simulink model "arduino_closed_loop_opcua"  (R2020b)
settings: Solver=FixedStepAuto  StartTime=0.0  StopTime=900  FixedStep=0.1  RelTol=1e-3
PreLoadFcn:
  | set_point=30;
  | kp=1.6;
  | ki=1/114.07;
libraries: slpidlib x1, realtime_pacer_lib x1
settings Model: Creator=Jonas  LastModifiedBy=MY DELL
settings SolverCC: AlgebraicLoopSolver=LineSearch
settings DataIOCC: ExternalInput=[uaClient]

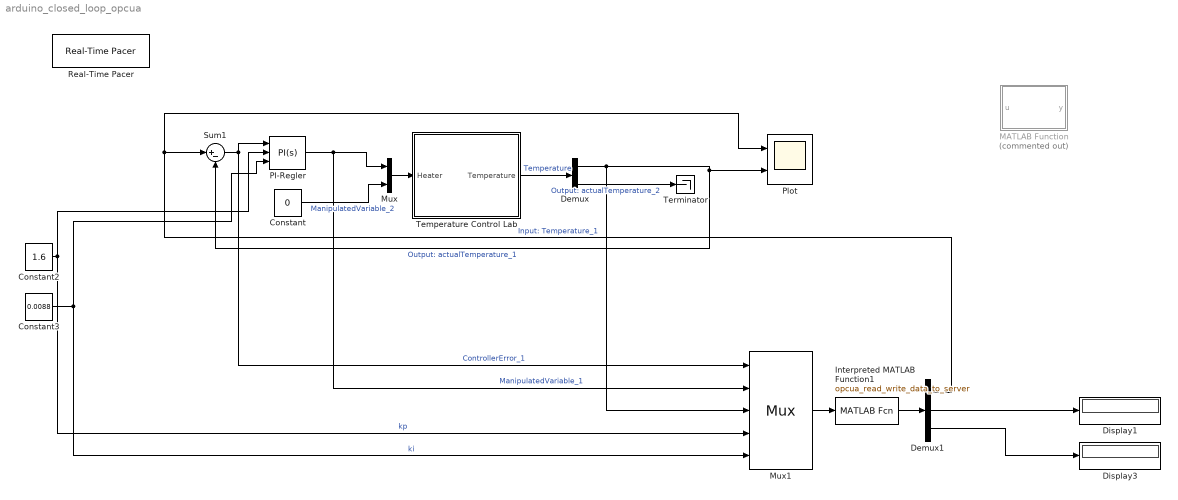
== system arduino_closed_loop_opcua ==
  Constant : Constant  Value=0
  Constant2 : Constant  Value=1.6
  Constant3 : Constant  Value=0.0088
  Demux : Demux  Outputs=2
  Demux1 : Demux  Outputs=3
  Display1 : Display
  Display3 : Display
  Interpreted MATLAB Function1 : MATLABFcn  MATLABFcn=opcua_read_write_data_to_server  OutputDimensions=3
  MATLAB Function : MATLAB Function  Commented=on  TreatAsAtomicUnit=on
  Mux : Mux  Inputs=2
  Mux1 : Mux  Inputs=5
      settings: DisplayOption=signals
  PI-Regler : slpidlib/PID Controller  Controller=PI  Form=Ideal  TimeDomain=Continuous-time  UseExternalTs=off  SampleTime=-1  IntegratorMethod=Forward Euler  FilterMethod=Forward Euler  ControllerParametersSource=external  P=1.6  I=0.0088  D=0  UseFilter=on  N=100  TunerSelectOption=Transfer Function Based (PID Tuner App)  ZeroCross=off  InitialConditionSource=internal  InitialConditionForIntegrator=0  InitialConditionForFilter=0  DifferentiatorICPrevScaledInput=0  ExternalReset=none  TrackingMode=off  Kt=1  LimitOutput=on  SatLimitsSource=internal  UpperSaturationLimit=80  LowerSaturationLimit=0  LinearizeAsGain=on  AntiWindupMode=none  Kb=1  POutMin=[]  POutMax=[]  IOutMin=[]  IOutMax=[]  DOutMin=[]  DOutMax=[]  NOutMin=[]  NOutMax=[]  SumOutMin=[]  SumOutMax=[]  SaturationOutMin=[]  SaturationOutMax=[]  PParamMin=[]  PParamMax=[]  IParamMin=[]  IParamMax=[]  DParamMin=[]  DParamMax=[]  NParamMin=[]  NParamMax=[]  KbParamMin=[]  KbParamMax=[]  KtParamMin=[]  KtParamMax=[]  KbOutMin=[]  KbOutMax=[]  KtOutMin=[]  KtOutMax=[]  IntegratorOutMin=[]  IntegratorOutMax=[]  FilterOutMin=[]  FilterOutMax=[]  SumI1OutMin=[]  SumI1OutMax=[]  SumI2OutMin=[]  SumI2OutMax=[]  SumI3OutMin=[]  SumI3OutMax=[]  SumI4OutMin=[]  SumI4OutMax=[]  SumDOutMin=[]  SumDOutMax=[]  DifferentiatorOutMin=[]  DifferentiatorOutMax=[]  FilterDiffOutCoefMin=[]  FilterDiffOutCoefMax=[]  ReciprocalOutMin=[]  ReciprocalOutMax=[]  SumDenOutMin=[]  SumDenOutMax=[]  SumNumOutMin=[]  SumNumOutMax=[]  DivideOutMin=[]  DivideOutMax=[]  UdiffTsProdOutMin=[]  UdiffTsProdOutMax=[]  NTsProdOutMin=[]  NTsProdOutMax=[]  UintegralTsProdOutMin=[]  UintegralTsProdOutMax=[]  UngainTsProdOutMin=[]  UngainTsProdOutMax=[]  IntegratorContinuousStateAttributes=''  IntegratorStateMustResolveToSignalObject=off  IntegratorRTWStateStorageClass=Auto  FilterContinuousStateAttributes=''  FilterStateMustResolveToSignalObject=off  FilterRTWStateStorageClass=Auto  ParallelPVariant=Passthrough  IdealPVariant=ExternalParameters  IVariant=ExternalParameters  DVariant=Disabled  IntegratorVariant=Continuous  SatVariant=Enabled  AWVariant=Passthrough  PCopyVariant=Disabled  TRVariant=Disabled  FdbkBlocksVariant=Forward  IdealPFdbkVariant=Disabled  SatFdbkVariant=Disabled  DerivativeFilterVariant=Disabled  NVariant=Disabled  NCopyVariant=Disabled_SignalSpec  FilterICVariant=Disabled  IntegratorICVariant=InternalICs  ExternalResetVariant=Disabled  TRSumVariant=Passthrough  SumFdbkVariant=Disabled  SumVariant=Sum_PI  TsampFilterVariant=InternalTs  TsampNgainVariant=Passthrough  TsampIntegralVariant=Passthrough  ExternalSaturationOutDataTypeStr=Inherit: Same as second input
  Plot : Scope  NumInputPorts=2
  Real-Time Pacer : realtime_pacer_lib/Real-Time Pacer  simTimePerRealTime=1
  Sum1 : Sum  Inputs=|+-
  Temperature Control Lab : Subsystem
  Terminator : Terminator
  wires:
  Sum1/1 -> PI-Regler/1, Mux1/1  "ControllerError_1"
  Demux1/1 -> Plot/1, Sum1/1  "Input: Temperature_1"
  PI-Regler/1 -> Mux1/2, Mux/1  "ManipulatedVariable_1"
  Demux/1 -> Mux1/3, Sum1/2, Plot/2  "Output: actualTemperature_1"
  Mux/1 -> Temperature Control Lab/1(Heater)
  Constant/1 -> Mux/2  "ManipulatedVariable_2"
  Temperature Control Lab/1(Temperature) -> Demux/1  "Temperature"
  Demux/2 -> Terminator/1  "Output: actualTemperature_2"
  Mux1/1 -> Interpreted MATLAB Function1/1
  Interpreted MATLAB Function1/1 -> Demux1/1
  Demux1/2 -> Display1/1
  Demux1/3 -> Display3/1
  Constant2/1 -> Mux1/4, PI-Regler/2  "kp"
  Constant3/1 -> Mux1/5, PI-Regler/3  "ki"

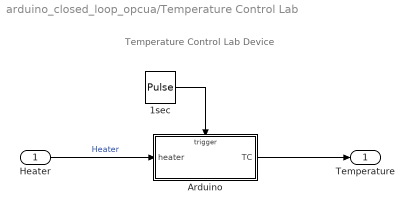
== system arduino_closed_loop_opcua/Temperature Control Lab ==
  note: Temperature Control Lab Device
  Heater : Inport
  1sec : DiscretePulseGenerator  PulseType=Time based  Period=1  PulseWidth=50
  Arduino : Subsystem  TreatAsAtomicUnit=on
  Temperature : Outport  VectorParamsAs1DForOutWhenUnconnected=off
  wires:
  1sec/1 -> Arduino/Trigger
  Arduino/1(TC) -> Temperature/1
  Heater/1 -> Arduino/1(heater)  "Heater"

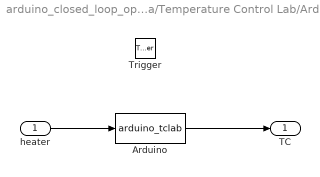
== system arduino_closed_loop_opcua/Temperature Control Lab/Arduino ==
  heater : Inport  LatchByDelayingOutsideSignal=on
  Trigger : TriggerPort  VariantControl=Variant
  Arduino : MATLABFcn  MATLABFcn=arduino_tclab
  TC : Outport  InitialOutput=[23 23]  VectorParamsAs1DForOutWhenUnconnected=off
  wires:
  heater/1 -> Arduino/1
  Arduino/1 -> TC/1

== matlab function arduino_closed_loop_opcua/MATLAB Function ==
  data: u input; y output
function y = opcua_read_write_data_to_server(u)

persistent uaClient heater_1 input_1 kp ki CO1 CE1

if (isempty(uaClient))
uaClient = opcua('localhost', 4840);
setSecurityModel(uaClient,'None');
connect(uaClient);
heater_1 = findNodeByName(uaClient.Namespace, 'Output: actualTemperature_1');
%heater_2 = findNodeByName(uaClient.Namespace, 'Output: actualTemperature_2');
input_1 = findNodeByName(uaClient.Namespace, 'Input: Temperature_1');
%input_2 = findNodeByName(uaClient.Namespace, 'Input: Temperature_2');
kp = findNodeByName(uaClient.Namespace, 'Proportional: Kp');
ki = findNodeByName(uaClient.Namespace, 'Integral: Ki');
CO1 = findNodeByName(uaClient.Namespace, 'ManipulatedVariable_1');
%CO2 = findNodeByName(uaClient.Namespace, 'ManipulatedVariable_2');
CE1 = findNodeByName(uaClient.Namespace, 'ControllerError_1');
%CE2 = findNodeByName(uaClient.Namespace, 'ControllerError_2');
y=[30;1.6;0.0088];%evt. auskommentieren
%writeValue(heater_1, 0);
%writeValue(heater_2, 0);

else
y=[30;1.6;0.0088];
writeValue(CE1, u(1));
writeValue(CO1, u(2));
%writeValue(CO2, u(3));
writeValue(heater_1, u(3));
%writeValue(heater_2, u(5));
writeValue(kp, u(4));
writeValue(ki, u(5));
[val1,ts1,qual1] = readValue(input_1);
[val2,ts2,qual2] = readValue(kp);
[val3,ts3,qual3] = readValue(ki);
y=[val1;val2;val3];
end

end
